simulink model "Lecture4_DiscretePID"  (R2020b)
settings: Solver=VariableStepAuto  StartTime=0.0  StopTime=10.0  RelTol=1e-3
values from neighbouring files (symbols this model uses):
  Gpd = [1 3 4]    [Lecture4_DiscretePID.m]
  Gpn = [10]    [Lecture4_DiscretePID.m]
  Kd = 1/2    (= 0.5)    [Assignment3.m]    (also in Lecture13_PolePlacement.m = -0.05; Lecture4_DiscretePID.m = 0.3)
  Ki = 1/2    (= 0.5)    [Assignment3.m]    (also in Assignment4.m = -K(3); Lecture13_PolePlacement.m = 0.0125; Lecture4_DiscretePID.m = 0.8)
  Kp = 1/2    (= 0.5)    [Assignment3.m]    (also in Lecture13_PolePlacement.m = -0.025; Lecture4_DiscretePID.m = 0.8)
  T = 1/((20*wc)/(2*pi))    (= 0.0010471975512)    [Assignment1.m]    (also in Assignment3.m = [1/(2.5*bw) 1/(10*bw) 1/(25*bw)]; Lecture15_DigitalLSF.m = 1 / ((25 * bandwidth(tf([10], [2 2 1])))); Lecture4_DiscretePID.m = 0.1)
settings Model: Creator=sebastian  LastModifiedBy=sebastian

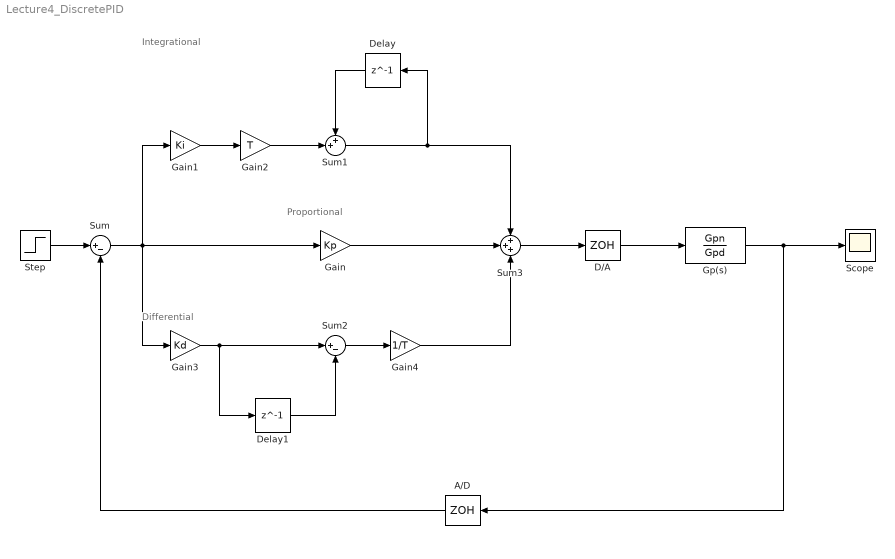
== system Lecture4_DiscretePID ==
  note: Integrational
  note: Differential
  note: Proportional
  A/D : ZeroOrderHold  SampleTime=T
  D/A : ZeroOrderHold  SampleTime=T
  Delay : Delay  DelayLength=1  SampleTime=T
  Delay1 : Delay  DelayLength=1  SampleTime=T
  Gain : Gain  Gain=Kp
  Gain1 : Gain  Gain=Ki
  Gain2 : Gain  Gain=T
  Gain3 : Gain  Gain=Kd
  Gain4 : Gain  Gain=1/T
  Gp(s) : TransferFcn  Numerator=Gpn  Denominator=Gpd
  Scope : Scope
  Step : Step  SampleTime=0
  Sum : Sum  Inputs=|+-
  Sum1 : Sum  Inputs=++|
  Sum2 : Sum  Inputs=|+-
  Sum3 : Sum  Inputs=+++
  wires:
  D/A/1 -> Gp(s)/1
  Gp(s)/1 -> A/D/1, Scope/1
  Step/1 -> Sum/1
  A/D/1 -> Sum/2
  Sum/1 -> Gain3/1, Gain1/1, Gain/1
  Gain1/1 -> Gain2/1
  Gain3/1 -> Sum2/1, Delay1/1
  Delay1/1 -> Sum2/2
  Sum2/1 -> Gain4/1
  Gain2/1 -> Sum1/2
  Delay/1 -> Sum1/1
  Sum1/1 -> Sum3/1, Delay/1
  Gain/1 -> Sum3/2
  Gain4/1 -> Sum3/3
  Sum3/1 -> D/A/1
